simulink model "JointSpaceControl_BestInertia"  (R2013a)
settings: Solver=ode3  StartTime=0.0  StopTime=sim_end  FixedStep=0.004  MaxStep=0.008  RelTol=1e-3
PreLoadFcn:
  | Initialization
InitFcn:
  | Initialization
values from neighbouring files (symbols this model uses):
  a_max = [27 27 27 27 27 27]    [Initialization.m]
  dq_0 = qd_actual.signals.values(1,:)    [Initialization.m]
  K_0 = [K0_11, zeros(3,3); zeros(3,3),omega_P_small^2*eye(3,3)]    [Initialization.m]    (also in Plot_PD_Estimation.m)
  K_1 = [K1_11, zeros(3,3); zeros(3,3),2*omega_D_small*eye(3,3)]    [Initialization.m]    (also in Plot_PD_Estimation.m)
  q_0 = q_actual.signals.values(1,:)    [Initialization.m]
  q_max = 2*pi*ones(1,6)    [Initialization.m]
  q_min = -2*pi*ones(1,6)    [Initialization.m]
  torque_max = [150 150 150 28 28 28]    [Initialization.m]
  v_max = 3.4*ones(1,6)    [Initialization.m]
libraries: dsparch4 x30, simulink x2
(part 1 of 3)
settings Model: Creator=kasiunia  LastModifiedBy=kasiunia

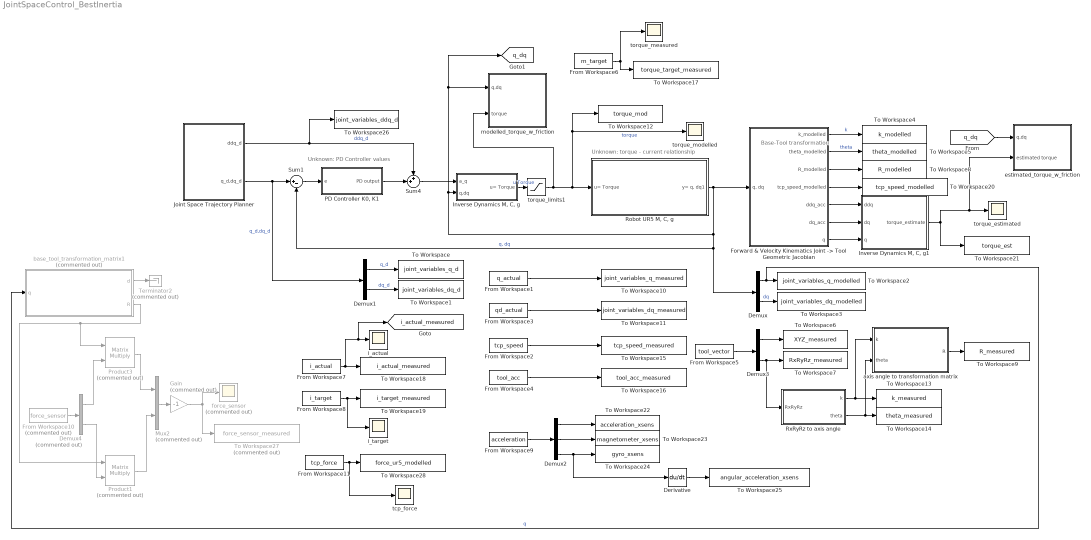
== system JointSpaceControl_BestInertia ==
  note: Base-Tool transformation
  note: Unknown: torque - current relationship
  note: Unknown: PD Controller values
  Demux : Demux  Outputs=[6 6]
  Demux1 : Demux  Outputs=[6 6]
  Demux2 : Demux  Outputs=[3 3 3]
  Demux3 : Demux  Outputs=[3 3]
  Demux4 : Demux  Commented=on  Outputs=[3 3 ]
  Derivative : Derivative
  "Forward & Velocity Kinematics Joint -> Tool Geometric Jacobian" : Subsystem
  From Workspace1 : FromWorkspace  VariableName=q_actual  SampleTime=0  OutputAfterFinalValue=Holding final value
  From Workspace10 : FromWorkspace  Commented=on  VariableName=force_sensor  SampleTime=0  OutputAfterFinalValue=Holding final value
  From Workspace11 : FromWorkspace  VariableName=tcp_force  SampleTime=0  OutputAfterFinalValue=Holding final value
  From Workspace2 : FromWorkspace  VariableName=tcp_speed  SampleTime=0  OutputAfterFinalValue=Setting to zero
  From Workspace3 : FromWorkspace  VariableName=qd_actual  SampleTime=0  OutputAfterFinalValue=Setting to zero
  From Workspace4 : FromWorkspace  VariableName=tool_acc  SampleTime=0  OutputAfterFinalValue=Setting to zero
  From Workspace5 : FromWorkspace  VariableName=tool_vector  SampleTime=0  OutputAfterFinalValue=Holding final value
  From Workspace6 : FromWorkspace  VariableName=m_target  SampleTime=0  OutputAfterFinalValue=Holding final value
  From Workspace7 : FromWorkspace  VariableName=i_actual  SampleTime=0  OutputAfterFinalValue=Holding final value
  From Workspace8 : FromWorkspace  VariableName=i_target  SampleTime=0  OutputAfterFinalValue=Holding final value
  From Workspace9 : FromWorkspace  VariableName=acceleration  SampleTime=0  OutputAfterFinalValue=Setting to zero
  Gain : Gain  Commented=on  Gain=-1
  "Inverse Dynamics M, C, g" : Subsystem
  "Inverse Dynamics M, C, g1" : Subsystem
  Joint Space Trajectory Planner : Subsystem
  Mux2 : Mux  Commented=on  Inputs=[3 3]
  "PD Controller K0, K1" : Subsystem
  Product1 : Product  Commented=on  Multiplication=Matrix(*)
  Product3 : Product  Commented=on  Multiplication=Matrix(*)
  "Robot UR5 M, C, g" : Subsystem
  RxRyRz to axis angle : MATLAB Function  TreatAsAtomicUnit=on
  Sum1 : Sum  Inputs=|+-
  Sum4 : Sum  Inputs=++|
  Terminator2 : Terminator  Commented=on
  To Workspace : ToWorkspace  VariableName=joint_variables_q_d  SampleTime=-1  SaveFormat=Timeseries
  To Workspace1 : ToWorkspace  VariableName=joint_variables_dq_d  SampleTime=-1  SaveFormat=Timeseries
  To Workspace10 : ToWorkspace  VariableName=joint_variables_q_measured  SampleTime=-1  SaveFormat=Timeseries
  To Workspace11 : ToWorkspace  VariableName=joint_variables_dq_measured  SampleTime=-1  SaveFormat=Timeseries
  To Workspace12 : ToWorkspace  VariableName=torque_mod  SampleTime=-1  SaveFormat=Timeseries
  To Workspace13 : ToWorkspace  VariableName=k_measured  SampleTime=-1  SaveFormat=Timeseries
  To Workspace14 : ToWorkspace  VariableName=theta_measured  SampleTime=-1  SaveFormat=Timeseries
  To Workspace15 : ToWorkspace  VariableName=tcp_speed_measured  SampleTime=-1  SaveFormat=Timeseries
  To Workspace16 : ToWorkspace  VariableName=tool_acc_measured  SampleTime=-1  SaveFormat=Timeseries
  To Workspace17 : ToWorkspace  VariableName=torque_target_measured  SampleTime=-1  SaveFormat=Timeseries
  To Workspace18 : ToWorkspace  VariableName=i_actual_measured  SampleTime=-1  SaveFormat=Timeseries
  To Workspace19 : ToWorkspace  VariableName=i_target_measured  SampleTime=-1  SaveFormat=Timeseries
  To Workspace2 : ToWorkspace  VariableName=joint_variables_q_modelled  SampleTime=-1  SaveFormat=Timeseries
  To Workspace20 : ToWorkspace  VariableName=tcp_speed_modelled  SampleTime=-1  SaveFormat=Timeseries
  To Workspace21 : ToWorkspace  VariableName=torque_est  SampleTime=-1  SaveFormat=Timeseries
  To Workspace22 : ToWorkspace  VariableName=acceleration_xsens  SampleTime=-1  SaveFormat=Timeseries
  To Workspace23 : ToWorkspace  VariableName=magnetometer_xsens  SampleTime=-1  SaveFormat=Timeseries
  To Workspace24 : ToWorkspace  VariableName=gyro_xsens  SampleTime=-1  SaveFormat=Timeseries
  To Workspace25 : ToWorkspace  VariableName=angular_acceleration_xsens  SampleTime=-1  SaveFormat=Timeseries
  To Workspace26 : ToWorkspace  VariableName=joint_variables_ddq_d  SampleTime=-1  SaveFormat=Timeseries
  To Workspace27 : ToWorkspace  Commented=on  VariableName=force_sensor_measured  SampleTime=-1  SaveFormat=Timeseries
  To Workspace28 : ToWorkspace  VariableName=force_ur5_modelled  SampleTime=-1  SaveFormat=Timeseries
  To Workspace3 : ToWorkspace  VariableName=joint_variables_dq_modelled  SampleTime=-1  SaveFormat=Timeseries
  To Workspace4 : ToWorkspace  VariableName=k_modelled  SampleTime=-1  SaveFormat=Timeseries
  To Workspace5 : ToWorkspace  VariableName=theta_modelled  SampleTime=-1  SaveFormat=Timeseries
  To Workspace6 : ToWorkspace  VariableName=XYZ_measured  SampleTime=-1  SaveFormat=Timeseries
  To Workspace7 : ToWorkspace  VariableName=RxRyRz_measured  SampleTime=-1  SaveFormat=Timeseries
  To Workspace8 : ToWorkspace  VariableName=R_modelled  SampleTime=-1  SaveFormat=Timeseries
  To Workspace9 : ToWorkspace  VariableName=R_measured  SampleTime=-1  SaveFormat=Timeseries
  axis angle to transformation matrix : MATLAB Function  TreatAsAtomicUnit=on
  base_tool_transformation_matrix1 : MATLAB Function  Commented=on  TreatAsAtomicUnit=on
  estimated_torque_w_friction : Subsystem
  force_sensor : Scope  Commented=on
      settings: ShowLegends=on  SaveName=ScopeData19
  i_actual : Scope
      settings: ShowLegends=on  TimeRange=25  YMin=-10  YMax=15  SaveName=ScopeData12
  i_target : Scope
      settings: SaveName=ScopeData13
  modelled_torque_w_friction : Subsystem
  tcp_force : Scope
      settings: SaveName=ScopeData20
  torque_estimated : Scope
      settings: ShowLegends=on  TimeRange=30  YMin=-2250  YMax=2250  SaveName=ScopeData15
  torque_limits1 : Saturate  UpperLimit=torque_max  LowerLimit=-torque_max
  torque_measured : Scope
      settings: ShowLegends=on  TimeRange=20.1629  YMin=-30  YMax=90  SaveName=ScopeData16
  torque_modelled : Scope
      settings: ShowLegends=on  TimeRange=20.1629  YMin=-2.5  YMax=55  SaveName=ScopeData17
  tag scope: i_actual_measured=global, q_dq=global
  wires:
  Joint Space Trajectory Planner/2(q_d,dq_d) -> Sum1/1, Demux1/1  "q_d,dq_d"
  Sum1/1 -> "PD Controller K0, K1"/1(e)
  "Robot UR5 M, C, g"/1("y= q, dq1") -> Sum1/2, Demux/1, [q_dq], modelled_torque_w_friction/1(q,dq), "Inverse Dynamics M, C, g"/2(q,dq), "Forward & Velocity Kinematics Joint -> Tool Geometric Jacobian"/1("q, dq")  "q, dq"
  Joint Space Trajectory Planner/1(ddq_d) -> Sum4/1, To Workspace26/1  "ddq_d"
  Demux1/1 -> To Workspace/1  "q_d"
  Demux1/2 -> To Workspace1/1  "dq_d"
  Demux/1 -> base_tool_transformation_matrix1/1(q), To Workspace2/1  "q"
  Demux/2 -> To Workspace3/1  "dq"
  From Workspace5/1 -> Demux3/1
  Demux3/1 -> To Workspace6/1
  Demux3/2 -> RxRyRz to axis angle/1(RxRyRz), To Workspace7/1
  "Forward & Velocity Kinematics Joint -> Tool Geometric Jacobian"/1(k_modelled) -> To Workspace4/1  "k"
  "Forward & Velocity Kinematics Joint -> Tool Geometric Jacobian"/2(theta_modelled) -> To Workspace5/1  "theta"
  RxRyRz to axis angle/1(k) -> axis angle to transformation matrix/1(k), To Workspace13/1
  RxRyRz to axis angle/2(theta) -> axis angle to transformation matrix/2(theta), To Workspace14/1
  "Forward & Velocity Kinematics Joint -> Tool Geometric Jacobian"/3(R_modelled) -> To Workspace8/1
  axis angle to transformation matrix/1(R) -> To Workspace9/1
  From Workspace2/1 -> To Workspace15/1
  From Workspace4/1 -> To Workspace16/1
  From Workspace6/1 -> torque_measured/1, To Workspace17/1
  From Workspace7/1 -> [i_actual_measured], i_actual/1, To Workspace18/1
  From Workspace8/1 -> i_target/1, To Workspace19/1
  "Forward & Velocity Kinematics Joint -> Tool Geometric Jacobian"/4(tcp_speed_modelled) -> To Workspace20/1
  "Forward & Velocity Kinematics Joint -> Tool Geometric Jacobian"/5(ddq_acc) -> "Inverse Dynamics M, C, g1"/1(ddq)
  "Forward & Velocity Kinematics Joint -> Tool Geometric Jacobian"/6(dq_acc) -> "Inverse Dynamics M, C, g1"/2(dq)
  "Inverse Dynamics M, C, g1"/1(torque_estimate) -> To Workspace21/1, estimated_torque_w_friction/2(estimated torque), torque_estimated/1
  "Forward & Velocity Kinematics Joint -> Tool Geometric Jacobian"/7(q) -> "Inverse Dynamics M, C, g1"/3(q)
  From Workspace9/1 -> Demux2/1
  Demux2/1 -> To Workspace22/1
  Demux2/2 -> To Workspace23/1
  Demux2/3 -> To Workspace24/1, Derivative/1
  Derivative/1 -> To Workspace25/1
  "Inverse Dynamics M, C, g"/1(u= Torque) -> torque_limits1/1  "u Torque"
  torque_limits1/1 -> modelled_torque_w_friction/2(torque), torque_modelled/1, To Workspace12/1, "Robot UR5 M, C, g"/1(u= Torque)  "torque"
  From Workspace1/1 -> To Workspace10/1
  From Workspace3/1 -> To Workspace11/1
  From Workspace11/1 -> tcp_force/1, To Workspace28/1
  [q_dq] -> estimated_torque_w_friction/1(q,dq)
  "PD Controller K0, K1"/1(PD output) -> Sum4/2
  Sum4/1 -> "Inverse Dynamics M, C, g"/1(a_q)
  base_tool_transformation_matrix1/1(d) -> Terminator2/1
  base_tool_transformation_matrix1/2(R) -> Product1/1, Product3/1
  From Workspace10/1 -> Demux4/1
  Mux2/1 -> Gain/1
  Product3/1 -> Mux2/1
  Demux4/2 -> Product1/2
  Demux4/1 -> Product3/2
  Product1/1 -> Mux2/2
  Gain/1 -> force_sensor/1, To Workspace27/1

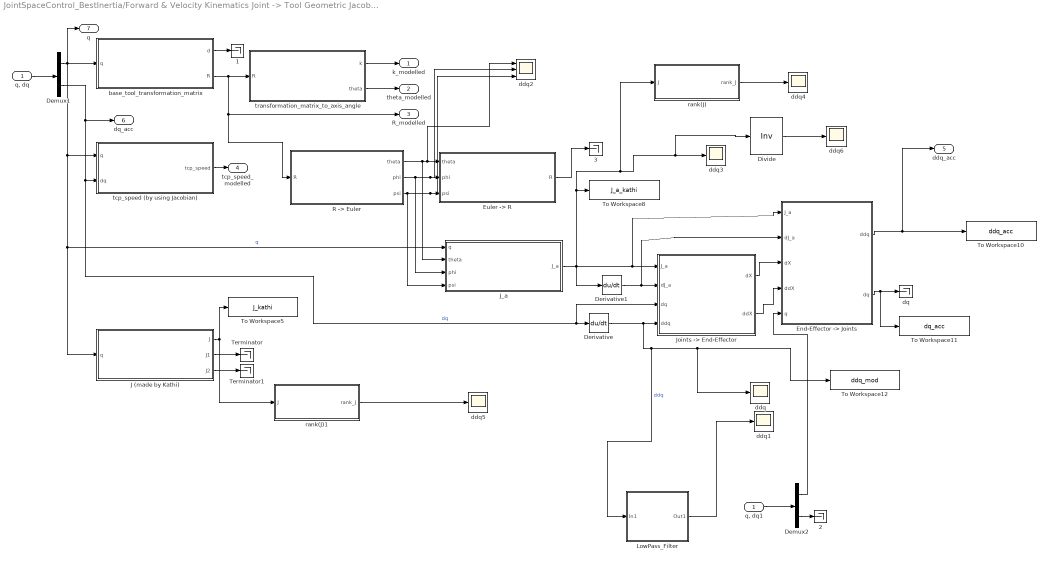
== system JointSpaceControl_BestInertia/Forward & Velocity Kinematics Joint -> Tool Geometric Jacobian ==
  "q, dq" : Inport
  1 : Terminator
  2 : Terminator
  3 : Terminator
  Demux1 : Demux  Outputs=[6 6]
  Demux2 : Demux  Outputs=[6 6]
  Derivative : Derivative
  Derivative1 : Derivative
  Divide : Product  Inputs=/  Multiplication=Matrix(*)
  "End-Effector -> Joints" : Subsystem
  "Euler -> R" : MATLAB Function  TreatAsAtomicUnit=on
  J (made by Kathi) : MATLAB Function  TreatAsAtomicUnit=on
  J_a : MATLAB Function  TreatAsAtomicUnit=on
  "Joints -> End-Effector" : Subsystem
  LowPass_Filter : Subsystem
  "R -> Euler" : MATLAB Function  TreatAsAtomicUnit=on
  Terminator : Terminator
  Terminator1 : Terminator
  To Workspace10 : ToWorkspace  VariableName=ddq_acc  SampleTime=-1  SaveFormat=Timeseries
  To Workspace11 : ToWorkspace  VariableName=dq_acc  SampleTime=-1  SaveFormat=Timeseries
  To Workspace12 : ToWorkspace  VariableName=ddq_mod  SampleTime=-1  SaveFormat=Timeseries
  To Workspace5 : ToWorkspace  VariableName=J_kathi  SampleTime=-1  SaveFormat=Timeseries
  To Workspace8 : ToWorkspace  VariableName=J_a_kathi  SampleTime=-1  SaveFormat=Timeseries
  base_tool_transformation_matrix : MATLAB Function  TreatAsAtomicUnit=on
  ddq{,1,3..6} (6 alike) : Scope
      ddq settings: ShowLegends=on  SaveName=ScopeData7
      ddq1 settings: ShowLegends=on  SaveName=ScopeData35
      ddq3 settings: ShowLegends=on  SaveName=ScopeData5
      ddq4 settings: ShowLegends=on  SaveName=ScopeData9
      ddq5 settings: ShowLegends=on  SaveName=ScopeData10
      ddq6 settings: ShowLegends=on  SaveName=ScopeData11
  ddq2 : Scope  NumInputPorts=3
      settings: ShowLegends=on  YMin=-5~-5~-5  YMax=5~5~5
  dq : Terminator
  "q, dq1" : InportShadow
  rank(J) : MATLAB Function  TreatAsAtomicUnit=on
  rank(J)1 : MATLAB Function  TreatAsAtomicUnit=on
  tcp_speed (by using Jacobian) : MATLAB Function  TreatAsAtomicUnit=on
  transformation_matrix_to_axis_angle : MATLAB Function  TreatAsAtomicUnit=on
  k_modelled : Outport
  theta_modelled : Outport  Port=2
  R_modelled : Outport  Port=3
  tcp_speed_modelled : Outport  Port=4
  ddq_acc : Outport  Port=5
  dq_acc : Outport  Port=6
  q : Outport  Port=7
  wires:
  "q, dq"/1 -> Demux1/1
  Demux1/1 -> q/1, J (made by Kathi)/1(q), J_a/1(q), tcp_speed (by using Jacobian)/1(q), base_tool_transformation_matrix/1(q)  "q"
  Demux1/2 -> dq_acc/1, "Joints -> End-Effector"/3(dq), Derivative/1, tcp_speed (by using Jacobian)/2(dq)  "dq"
  base_tool_transformation_matrix/2(R) -> transformation_matrix_to_axis_angle/1(R), "R -> Euler"/1(R), R_modelled/1
  transformation_matrix_to_axis_angle/1(k) -> k_modelled/1
  transformation_matrix_to_axis_angle/2(theta) -> theta_modelled/1
  J (made by Kathi)/1(J) -> To Workspace5/1, rank(J)1/1(J)
  tcp_speed (by using Jacobian)/1(tcp_speed) -> tcp_speed_modelled/1
  "R -> Euler"/3(psi) -> J_a/4(psi), ddq2/3, "Euler -> R"/3(psi)
  "R -> Euler"/2(phi) -> J_a/3(phi), ddq2/2, "Euler -> R"/2(phi)
  "R -> Euler"/1(theta) -> J_a/2(theta), ddq2/1, "Euler -> R"/1(theta)
  base_tool_transformation_matrix/1(d) -> 1/1
  J_a/1(J_a) -> "Joints -> End-Effector"/1(J_a), "End-Effector -> Joints"/1(J_a), rank(J)/1(J), Divide/1, ddq3/1, To Workspace8/1, Derivative1/1
  Derivative/1 -> "Joints -> End-Effector"/4(ddq), LowPass_Filter/1(In1), ddq/1, To Workspace12/1  "ddq"
  "Joints -> End-Effector"/2(ddX) -> "End-Effector -> Joints"/4(ddX)
  "Joints -> End-Effector"/1(dX) -> "End-Effector -> Joints"/3(dX)
  Derivative1/1 -> "Joints -> End-Effector"/2(dJ_a), "End-Effector -> Joints"/2(dJ_a)
  "End-Effector -> Joints"/2(dq) -> To Workspace11/1, dq/1
  J (made by Kathi)/2(J1) -> Terminator/1
  J (made by Kathi)/3(J2) -> Terminator1/1
  "End-Effector -> Joints"/1(ddq) -> ddq_acc/1, To Workspace10/1
  "q, dq1"/1 -> Demux2/1
  Demux2/2 -> 2/1
  Demux2/1 -> "End-Effector -> Joints"/5(q)
  "Euler -> R"/1(R) -> 3/1
  LowPass_Filter/1(Out1) -> ddq1/1
  rank(J)/1(rank_J) -> ddq4/1
  rank(J)1/1(rank_J) -> ddq5/1
  Divide/1 -> ddq6/1

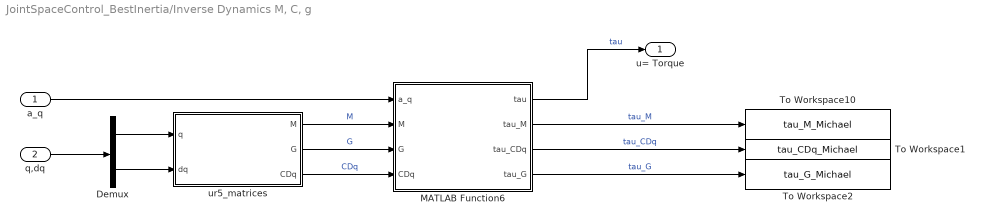
== system JointSpaceControl_BestInertia/Inverse Dynamics M, C, g ==
  a_q : Inport
  q,dq : Inport  Port=2
  Demux : Demux  Outputs=[6 6]
  MATLAB Function6 : MATLAB Function  TreatAsAtomicUnit=on
  To Workspace1 : ToWorkspace  VariableName=tau_CDq_Michael  SampleTime=-1  SaveFormat=Timeseries
  To Workspace10 : ToWorkspace  VariableName=tau_M_Michael  SampleTime=-1  SaveFormat=Timeseries
  To Workspace2 : ToWorkspace  VariableName=tau_G_Michael  SampleTime=-1  SaveFormat=Timeseries
  ur5_matrices : MATLAB Function  TreatAsAtomicUnit=on
  u= Torque : Outport
  wires:
  ur5_matrices/1(M) -> MATLAB Function6/2(M)  "M"
  ur5_matrices/3(CDq) -> MATLAB Function6/4(CDq)  "CDq"
  a_q/1 -> MATLAB Function6/1(a_q)
  Demux/1 -> ur5_matrices/1(q)
  Demux/2 -> ur5_matrices/2(dq)
  q,dq/1 -> Demux/1
  MATLAB Function6/1(tau) -> u= Torque/1  "tau"
  MATLAB Function6/2(tau_M) -> To Workspace10/1  "tau_M"
  MATLAB Function6/3(tau_CDq) -> To Workspace1/1  "tau_CDq"
  MATLAB Function6/4(tau_G) -> To Workspace2/1  "tau_G"
  ur5_matrices/2(G) -> MATLAB Function6/3(G)  "G"

== system JointSpaceControl_BestInertia/Inverse Dynamics M, C, g1 ==
  ddq : Inport
  dq : Inport  Port=2
  q : Inport  Port=3
  ur5_invDynamics : MATLAB Function  TreatAsAtomicUnit=on
  ur5_matrices : MATLAB Function  TreatAsAtomicUnit=on
  torque_estimate : Outport
  wires:
  ur5_invDynamics/1(tau) -> torque_estimate/1  "tau"
  ddq/1 -> ur5_invDynamics/1(a_q)
  ur5_matrices/3(CDq) -> ur5_invDynamics/4(CDq)
  ur5_matrices/2(G) -> ur5_invDynamics/3(G)
  ur5_matrices/1(M) -> ur5_invDynamics/2(M)
  q/1 -> ur5_matrices/1(q)
  dq/1 -> ur5_matrices/2(dq)

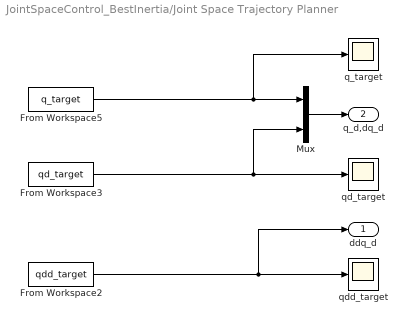
== system JointSpaceControl_BestInertia/Joint Space Trajectory Planner ==
  From Workspace2 : FromWorkspace  VariableName=qdd_target  SampleTime=0  OutputAfterFinalValue=Setting to zero
  From Workspace3 : FromWorkspace  VariableName=qd_target  SampleTime=0  OutputAfterFinalValue=Setting to zero
  From Workspace5 : FromWorkspace  VariableName=q_target  SampleTime=0  OutputAfterFinalValue=Holding final value
  Mux : Mux  Inputs=[6 6]
  q_target : Scope
      settings: ShowLegends=on
  qd_target : Scope
      settings: ShowLegends=on  SaveName=ScopeData2
  qdd_target : Scope
      settings: ShowLegends=on  SaveName=ScopeData3
  ddq_d : Outport
  q_d,dq_d : Outport  Port=2
  wires:
  Mux/1 -> q_d,dq_d/1
  From Workspace5/1 -> Mux/1, q_target/1
  From Workspace3/1 -> Mux/2, qd_target/1
  From Workspace2/1 -> ddq_d/1, qdd_target/1

== system JointSpaceControl_BestInertia/PD Controller K0, K1 ==
  e : Inport
  Demux : Demux  Outputs=[6 6]
  Gain : Gain  Gain=K_0  Multiplication=Matrix(K*u) (u vector)
  Gain1 : Gain  Gain=K_1  Multiplication=Matrix(K*u) (u vector)
  Sum : Sum  Inputs=|++
  PD output : Outport
  wires:
  e/1 -> Demux/1
  Sum/1 -> PD output/1
  Demux/1 -> Gain/1  "e_q = q_d - q"
  Demux/2 -> Gain1/1  "e_dq = dq_d - dq"
  Gain1/1 -> Sum/2
  Gain/1 -> Sum/1

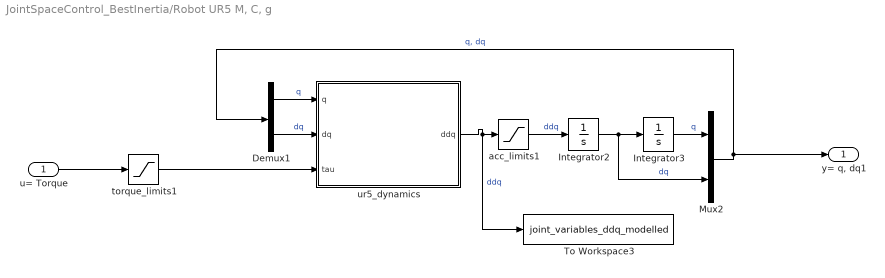
== system JointSpaceControl_BestInertia/Robot UR5 M, C, g ==
  u= Torque : Inport
  Demux1 : Demux  Outputs=[6 6]
  Integrator2 : Integrator  InitialCondition=[dq_0]  LimitOutput=on  UpperSaturationLimit=v_max  LowerSaturationLimit=-v_max  ContinuousStateAttributes='velocity'
  Integrator3 : Integrator  InitialCondition=[q_0]  LimitOutput=on  UpperSaturationLimit=q_max  LowerSaturationLimit=q_min  ContinuousStateAttributes='position'
  Mux2 : Mux  Inputs=[6 6]
  To Workspace3 : ToWorkspace  VariableName=joint_variables_ddq_modelled  SampleTime=-1  SaveFormat=Timeseries
  acc_limits1 : Saturate  UpperLimit=a_max  LowerLimit=-a_max
  torque_limits1 : Saturate  UpperLimit=torque_max  LowerLimit=-torque_max
  ur5_dynamics : MATLAB Function  TreatAsAtomicUnit=on
  "y= q, dq1" : Outport
  wires:
  ur5_dynamics/1(ddq) -> To Workspace3/1, acc_limits1/1  "ddq"
  Integrator2/1 -> Integrator3/1, Mux2/2  "dq"
  Integrator3/1 -> Mux2/1  "q"
  Mux2/1 -> "y= q, dq1"/1, Demux1/1  "q, dq"
  Demux1/1 -> ur5_dynamics/1(q)  "q"
  Demux1/2 -> ur5_dynamics/2(dq)  "dq"
  acc_limits1/1 -> Integrator2/1  "ddq"
  torque_limits1/1 -> ur5_dynamics/3(tau)
  u= Torque/1 -> torque_limits1/1

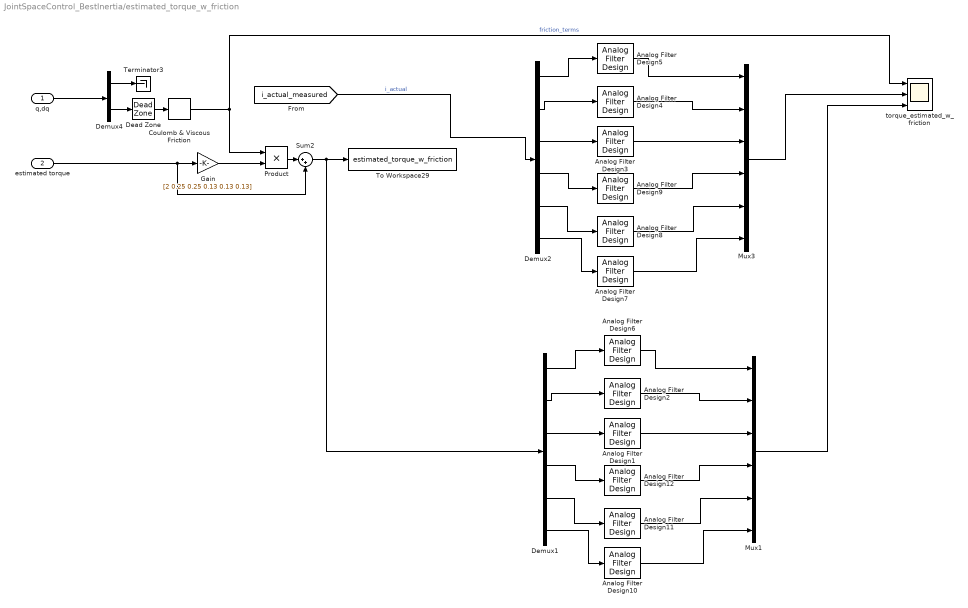
== system JointSpaceControl_BestInertia/estimated_torque_w_friction ==
  q,dq : Inport
  estimated torque : Inport  Port=2
  Analog Filter Design{1..12} (12 alike) : dsparch4/Analog Filter Design  method=Butterworth  filttype=Lowpass  N=10  Wlo=30  Whi=80  Rp=2  Rs=40
  Coulomb & Viscous Friction : simulink/Discontinuities/Coulomb & Viscous Friction  offset=1  gain=1
  Dead Zone : DeadZone  LowerValue=-0.02  UpperValue=0.02  SaturateOnIntegerOverflow=on
  Demux1 : Demux  Outputs=[1 1 1 1 1 1]
  Demux2 : Demux  Outputs=[1 1 1 1 1 1]
  Demux4 : Demux  Outputs=[6 6]
  Gain : Gain  Gain=[2 0.25 0.25 0.13 0.13 0.13]
  Mux1 : Mux  Inputs=[1 1 1 1 1 1]
  Mux3 : Mux  Inputs=[1 1 1 1 1 1]
  Product : Product
  Sum2 : Sum  Inputs=|++
  Terminator3 : Terminator
  To Workspace29 : ToWorkspace  VariableName=estimated_torque_w_friction  SampleTime=-1  SaveFormat=Timeseries
  torque_estimated_w_friction : Scope  NumInputPorts=3
      settings: ShowLegends=on  TimeRange=25  YMin=-2.25~-2~-40  YMax=2.25~6.5~80  SaveName=ScopeData18
  wires:
  estimated torque/1 -> Gain/1, Sum2/2
  q,dq/1 -> Demux4/1
  Demux4/2 -> Dead Zone/1
  Product/1 -> Sum2/1
  Dead Zone/1 -> Coulomb & Viscous Friction/1
  Sum2/1 -> Demux1/1, To Workspace29/1
  Gain/1 -> Product/2
  Coulomb & Viscous Friction/1 -> torque_estimated_w_friction/1, Product/1  "friction_terms"
  Demux4/1 -> Terminator3/1
  Demux2/1 -> Analog Filter Design5/1
  Demux2/2 -> Analog Filter Design4/1
  Demux2/3 -> Analog Filter Design3/1
  Analog Filter Design5/1 -> Mux3/1
  Analog Filter Design4/1 -> Mux3/2
  Analog Filter Design3/1 -> Mux3/3
  [i_actual_measured] -> Demux2/1  "i_actual"
  Mux3/1 -> torque_estimated_w_friction/2
  Demux2/4 -> Analog Filter Design9/1
  Demux2/5 -> Analog Filter Design8/1
  Demux2/6 -> Analog Filter Design7/1
  Analog Filter Design9/1 -> Mux3/4
  Analog Filter Design8/1 -> Mux3/5
  Analog Filter Design7/1 -> Mux3/6
  Demux1/1 -> Analog Filter Design6/1
  Demux1/2 -> Analog Filter Design2/1
  Demux1/3 -> Analog Filter Design1/1
  Analog Filter Design6/1 -> Mux1/1
  Analog Filter Design2/1 -> Mux1/2
  Analog Filter Design1/1 -> Mux1/3
  Demux1/4 -> Analog Filter Design12/1
  Demux1/5 -> Analog Filter Design11/1
  Demux1/6 -> Analog Filter Design10/1
  Analog Filter Design12/1 -> Mux1/4
  Analog Filter Design11/1 -> Mux1/5
  Analog Filter Design10/1 -> Mux1/6
  Mux1/1 -> torque_estimated_w_friction/3

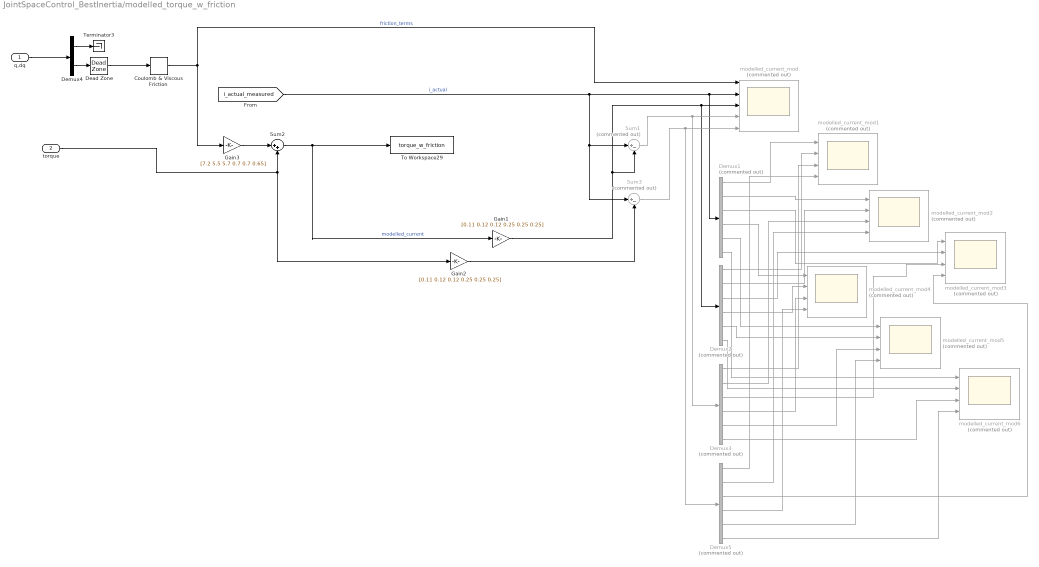
== system JointSpaceControl_BestInertia/modelled_torque_w_friction ==
  q,dq : Inport
  torque : Inport  Port=2
  Coulomb & Viscous Friction : simulink/Discontinuities/Coulomb & Viscous Friction  offset=1  gain=1
  Dead Zone : DeadZone  LowerValue=-0.02  UpperValue=0.02  SaturateOnIntegerOverflow=on
  Demux{1..3,5} (4 alike) : Demux  Commented=on  Outputs=[1 1 1 1 1 1]
  Demux4 : Demux  Outputs=[6 6]
  Gain1 : Gain  Gain=[0.11 0.12 0.12 0.25 0.25 0.25]
  Gain2 : Gain  Gain=[0.11 0.12 0.12 0.25 0.25 0.25]
  Gain3 : Gain  Gain=[7.2 5.5 5.7 0.7 0.7 0.65]
  Sum1 : Sum  Commented=on  Inputs=|+-
  Sum2 : Sum  Inputs=|++
  Sum3 : Sum  Commented=on  Inputs=|+-
  Terminator3 : Terminator
  To Workspace29 : ToWorkspace  VariableName=torque_w_friction  SampleTime=-1  SaveFormat=Timeseries
  modelled_current_mod : Scope  Commented=on  NumInputPorts=5
      settings: ShowLegends=on  TimeRange=15.704  YMin=-2.5~-2.5~-5~-5~-5  YMax=2.25~7.5~60~5~5  SaveName=ScopeData18
  modelled_current_mod{1..6} (6 alike) : Scope  Commented=on  NumInputPorts=4
      modelled_current_mod1 settings: ShowLegends=on  TimeRange=15.704  YMin=-2.5~-2.5~-5~-5  YMax=2.25~7.5~60~5  SaveName=ScopeData27
      modelled_current_mod2 settings: ShowLegends=on  TimeRange=15.704  YMin=-2.5~-2.5~-5~-5  YMax=2.25~7.5~60~5  SaveName=ScopeData28
      modelled_current_mod3 settings: ShowLegends=on  TimeRange=15.704  YMin=-2.5~-2.5~-5~-5  YMax=2.25~7.5~60~5  SaveName=ScopeData30
      modelled_current_mod4 settings: ShowLegends=on  TimeRange=15.704  YMin=-2.5~-2.5~-5~-5  YMax=2.25~7.5~60~5  SaveName=ScopeData31
      modelled_current_mod5 settings: ShowLegends=on  TimeRange=15.704  YMin=-2.5~-2.5~-5~-5  YMax=2.25~7.5~60~5  SaveName=ScopeData32
      modelled_current_mod6 settings: ShowLegends=on  TimeRange=15.704  YMin=-2.5~-2.5~-5~-5  YMax=2.25~7.5~60~5  SaveName=ScopeData33
  wires:
  [i_actual_measured] -> Sum3/1, Sum1/1, Demux1/1, modelled_current_mod/2  "i_actual"
  Demux4/1 -> Terminator3/1
  Coulomb & Viscous Friction/1 -> Gain3/1, modelled_current_mod/1  "friction_terms"
  Sum2/1 -> Gain1/1, To Workspace29/1  "modelled_current"
  Dead Zone/1 -> Coulomb & Viscous Friction/1
  Demux4/2 -> Dead Zone/1
  q,dq/1 -> Demux4/1
  Gain1/1 -> Sum1/2, Demux2/1, modelled_current_mod/3
  Sum1/1 -> Demux3/1, modelled_current_mod/4
  Sum3/1 -> Demux5/1, modelled_current_mod/5
  torque/1 -> Gain2/1, Sum2/2
  Gain2/1 -> Sum3/2
  Demux1/1 -> modelled_current_mod1/1
  Demux1/2 -> modelled_current_mod2/1
  Demux1/3 -> modelled_current_mod3/1
  Demux1/4 -> modelled_current_mod4/1
  Demux1/5 -> modelled_current_mod5/1
  Demux1/6 -> modelled_current_mod6/1
  Demux2/1 -> modelled_current_mod1/2
  Demux2/2 -> modelled_current_mod2/2
  Demux2/3 -> modelled_current_mod3/2
  Demux2/4 -> modelled_current_mod4/2
  Demux2/5 -> modelled_current_mod5/2
  Demux2/6 -> modelled_current_mod6/2
  Demux3/1 -> modelled_current_mod1/3
  Demux3/2 -> modelled_current_mod2/3
  Demux3/3 -> modelled_current_mod3/3
  Demux3/4 -> modelled_current_mod4/3
  Demux3/5 -> modelled_current_mod5/3
  Demux3/6 -> modelled_current_mod6/3
  Demux5/1 -> modelled_current_mod1/4
  Demux5/2 -> modelled_current_mod2/4
  Demux5/3 -> modelled_current_mod3/4
  Demux5/4 -> modelled_current_mod4/4
  Demux5/5 -> modelled_current_mod5/4
  Demux5/6 -> modelled_current_mod6/4
  Gain3/1 -> Sum2/1

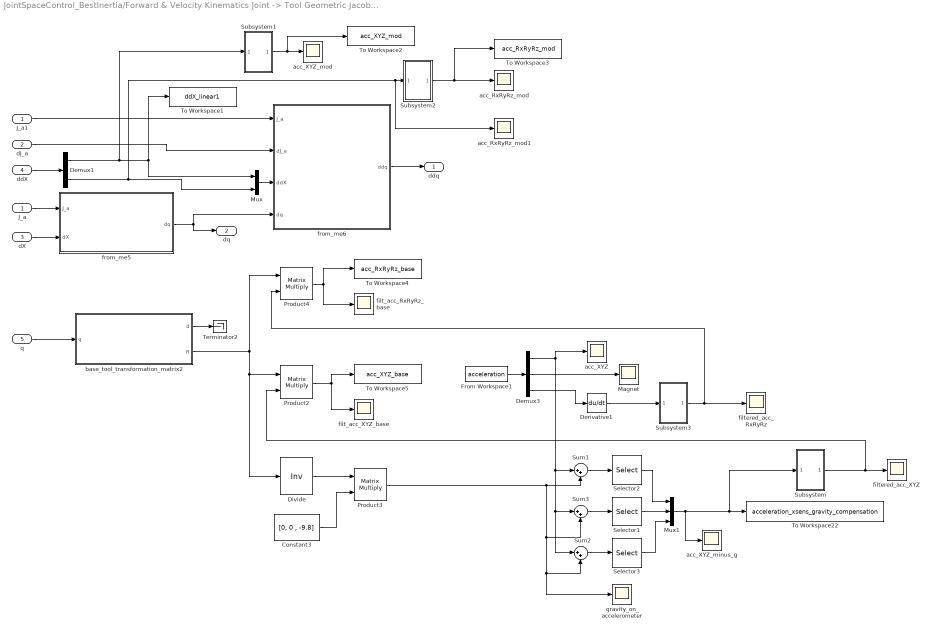
== system JointSpaceControl_BestInertia/Forward & Velocity Kinematics Joint -> Tool Geometric Jacobian/End-Effector -> Joints ==
  J_a : Inport
  dJ_a : Inport  Port=2
  dX : Inport  Port=3
  ddX : Inport  Port=4
  q : Inport  Port=5
  Constant3 : Constant  Value=[0, 0 , -9.8]
  Demux1 : Demux  Outputs=[3 3]
  Demux3 : Demux  Outputs=[3 3 3]
  Derivative1 : Derivative
  Divide : Product  Inputs=/  Multiplication=Matrix(*)
  From Workspace1 : FromWorkspace  VariableName=acceleration  SampleTime=0  OutputAfterFinalValue=Setting to zero
  J_a1 : InportShadow
  Magnet : Scope
      settings: ShowLegends=on  SaveName=ScopeData22
  Mux : Mux  Inputs=[3 3]
  Mux1 : Mux  Inputs=[1 1 1]
  Product2 : Product  Multiplication=Matrix(*)
  Product3 : Product  Multiplication=Matrix(*)
  Product4 : Product  Multiplication=Matrix(*)
  Selector1 : Selector  InputPortWidth=3  IndexOptions=Index vector (dialog)  Indices=[2]  OutputSizes=1
  Selector2 : Selector  InputPortWidth=3  IndexOptions=Index vector (dialog)  Indices=[1]  OutputSizes=1
  Selector3 : Selector  InputPortWidth=3  IndexOptions=Index vector (dialog)  Indices=[3]  OutputSizes=1
  Subsystem : Subsystem
  Subsystem1 : Subsystem
  Subsystem2 : Subsystem
  Subsystem3 : Subsystem
  Sum1 : Sum  Inputs=|++
  Sum2 : Sum  Inputs=|++
  Sum3 : Sum  Inputs=|++
  Terminator2 : Terminator
  To Workspace1 : ToWorkspace  VariableName=ddX_linear1  SampleTime=-1  SaveFormat=Timeseries
  To Workspace2 : ToWorkspace  VariableName=acc_XYZ_mod  SampleTime=-1  SaveFormat=Timeseries
  To Workspace22 : ToWorkspace  VariableName=acceleration_xsens_gravity_compensation  SampleTime=-1  SaveFormat=Timeseries
  To Workspace3 : ToWorkspace  VariableName=acc_RxRyRz_mod  SampleTime=-1  SaveFormat=Timeseries
  To Workspace4 : ToWorkspace  VariableName=acc_RxRyRz_base  SampleTime=-1  SaveFormat=Timeseries
  To Workspace5 : ToWorkspace  VariableName=acc_XYZ_base  SampleTime=-1  SaveFormat=Timeseries
  acc_RxRyRz_mod : Scope
      settings: ShowLegends=on  YMin=-3  YMax=3.5  SaveName=ScopeData34
  acc_RxRyRz_mod1 : Scope
      settings: ShowLegends=on  YMin=-3  YMax=3.5  SaveName=ScopeData6
  acc_XYZ : Scope
      settings: ShowLegends=on  YMin=-10  YMax=17.5  SaveName=ScopeData23
  acc_XYZ_minus_g : Scope
      settings: ShowLegends=on  YMin=-2.25  YMax=3  SaveName=ScopeData24
  acc_XYZ_mod : Scope
      settings: ShowLegends=on  YMin=-3  YMax=3.5  SaveName=ScopeData4
  base_tool_transformation_matrix2 : MATLAB Function  TreatAsAtomicUnit=on
  filt_acc_RxRyRz_base : Scope
      settings: ShowLegends=on  YMin=-3  YMax=3.5  SaveName=ScopeData21
  filt_acc_XYZ_base : Scope
      settings: ShowLegends=on  YMin=-3  YMax=3.5  SaveName=ScopeData8
  filtered_acc_RxRyRz : Scope
      settings: ShowLegends=on  SaveName=ScopeData29
  filtered_acc_XYZ : Scope
      settings: ShowLegends=on  YMin=-3  YMax=3.5  SaveName=ScopeData25
  from_me5 : MATLAB Function  TreatAsAtomicUnit=on
  from_me6 : MATLAB Function  TreatAsAtomicUnit=on
  gravity_on_accelerometer : Scope
      settings: ShowLegends=on  YMin=-6  YMax=9  SaveName=ScopeData14
  ddq : Outport
  dq : Outport  Port=2
  wires:
  from_me6/1(ddq) -> ddq/1
  J_a/1 -> from_me5/1(J_a)
  J_a1/1 -> from_me6/1(J_a)
  dJ_a/1 -> from_me6/2(dJ_a)
  dX/1 -> from_me5/2(dX)
  from_me5/1(dq) -> dq/1, from_me6/4(dq)
  Mux/1 -> from_me6/3(ddX)
  ddX/1 -> Demux1/1
  From Workspace1/1 -> Demux3/1
  Demux3/2 -> Magnet/1
  Demux3/3 -> Derivative1/1
  Demux3/1 -> Sum3/1, Sum2/1, Sum1/1, acc_XYZ/1
  Mux1/1 -> Subsystem/1(In1), To Workspace22/1, acc_XYZ_minus_g/1
  Sum1/1 -> Selector2/1
  Selector2/1 -> Mux1/1
  Sum2/1 -> Selector3/1
  Sum3/1 -> Selector1/1
  Divide/1 -> Product3/1
  Constant3/1 -> Product3/2
  base_tool_transformation_matrix2/2(R) -> Product4/1, Divide/1, Product2/1
  Product3/1 -> gravity_on_accelerometer/1, Sum2/2, Sum3/2, Sum1/2
  q/1 -> base_tool_transformation_matrix2/1(q)
  Selector1/1 -> Mux1/2
  Selector3/1 -> Mux1/3
  Demux1/1 -> Subsystem1/1(In1), To Workspace1/1, Mux/1
  Demux1/2 -> acc_RxRyRz_mod1/1, Subsystem2/1(In1), Mux/2
  base_tool_transformation_matrix2/1(d) -> Terminator2/1
  Subsystem/1(Out1) -> Product2/2, filtered_acc_XYZ/1
  Subsystem1/1(Out1) -> To Workspace2/1, acc_XYZ_mod/1
  Subsystem2/1(Out1) -> To Workspace3/1, acc_RxRyRz_mod/1
  Product4/1 -> To Workspace4/1, filt_acc_RxRyRz_base/1
  Product2/1 -> To Workspace5/1, filt_acc_XYZ_base/1
  Subsystem3/1(Out1) -> Product4/2, filtered_acc_RxRyRz/1
  Derivative1/1 -> Subsystem3/1(In1)

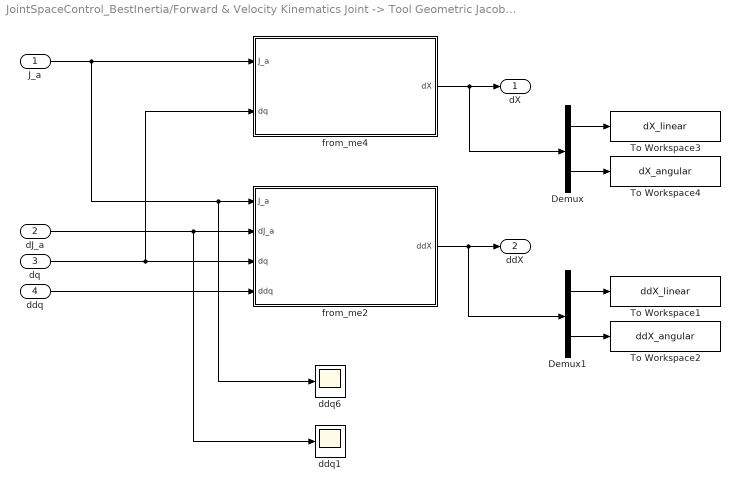
== system JointSpaceControl_BestInertia/Forward & Velocity Kinematics Joint -> Tool Geometric Jacobian/Joints -> End-Effector ==
  J_a : Inport
  dJ_a : Inport  Port=2
  dq : Inport  Port=3
  ddq : Inport  Port=4
  Demux : Demux  Outputs=[3 3]
  Demux1 : Demux  Outputs=[3 3]
  To Workspace1 : ToWorkspace  VariableName=ddX_linear  SampleTime=-1  SaveFormat=Timeseries
  To Workspace2 : ToWorkspace  VariableName=ddX_angular  SampleTime=-1  SaveFormat=Timeseries
  To Workspace3 : ToWorkspace  VariableName=dX_linear  SampleTime=-1  SaveFormat=Timeseries
  To Workspace4 : ToWorkspace  VariableName=dX_angular  SampleTime=-1  SaveFormat=Timeseries
  ddq1 : Scope
      settings: ShowLegends=on  SaveName=ScopeData36
  ddq6 : Scope
      settings: ShowLegends=on  SaveName=ScopeData26
  from_me2 : MATLAB Function  TreatAsAtomicUnit=on
  from_me4 : MATLAB Function  TreatAsAtomicUnit=on
  dX : Outport
  ddX : Outport  Port=2
  wires:
  from_me4/1(dX) -> Demux/1, dX/1
  from_me2/1(ddX) -> Demux1/1, ddX/1
  J_a/1 -> ddq6/1, from_me2/1(J_a), from_me4/1(J_a)
  dJ_a/1 -> ddq1/1, from_me2/2(dJ_a)
  dq/1 -> from_me4/2(dq), from_me2/3(dq)
  ddq/1 -> from_me2/4(ddq)
  Demux/1 -> To Workspace3/1
  Demux/2 -> To Workspace4/1
  Demux1/1 -> To Workspace1/1
  Demux1/2 -> To Workspace2/1

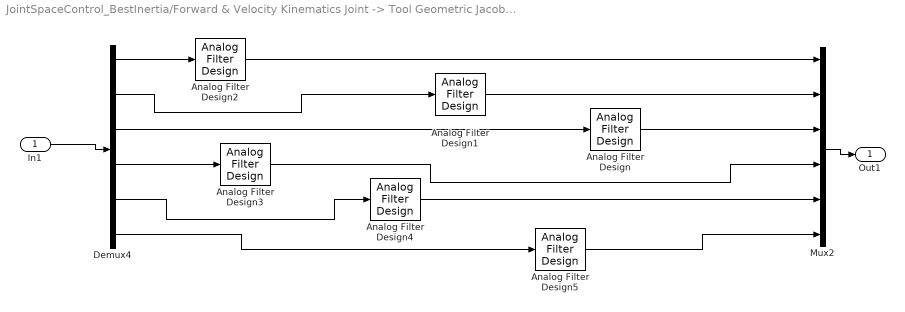
== system JointSpaceControl_BestInertia/Forward & Velocity Kinematics Joint -> Tool Geometric Jacobian/LowPass_Filter ==
  In1 : Inport
  Analog Filter Design{,1..5} (6 alike) : dsparch4/Analog Filter Design  method=Butterworth  filttype=Lowpass  N=3  Wlo=30  Whi=80  Rp=2  Rs=40
  Demux4 : Demux  Outputs=[1 1 1 1 1 1]
  Mux2 : Mux  Inputs=[1 1 1 1 1 1]
  Out1 : Outport
  wires:
  Mux2/1 -> Out1/1
  Analog Filter Design/1 -> Mux2/3
  Analog Filter Design1/1 -> Mux2/2
  Analog Filter Design2/1 -> Mux2/1
  Demux4/3 -> Analog Filter Design/1
  Demux4/2 -> Analog Filter Design1/1
  Demux4/1 -> Analog Filter Design2/1
  In1/1 -> Demux4/1
  Demux4/4 -> Analog Filter Design3/1
  Analog Filter Design3/1 -> Mux2/4
  Demux4/5 -> Analog Filter Design4/1
  Analog Filter Design4/1 -> Mux2/5
  Demux4/6 -> Analog Filter Design5/1
  Analog Filter Design5/1 -> Mux2/6

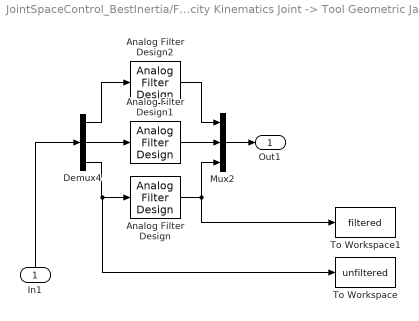
== system JointSpaceControl_BestInertia/Forward & Velocity Kinematics Joint -> Tool Geometric Jacobian/End-Effector -> Joints/Subsystem ==
  In1 : Inport
  Analog Filter Design : dsparch4/Analog Filter Design  method=Butterworth  filttype=Lowpass  N=8  Wlo=30  Whi=80  Rp=2  Rs=40
  Analog Filter Design1 : dsparch4/Analog Filter Design  method=Butterworth  filttype=Lowpass  N=8  Wlo=30  Whi=80  Rp=2  Rs=40
  Analog Filter Design2 : dsparch4/Analog Filter Design  method=Butterworth  filttype=Lowpass  N=8  Wlo=30  Whi=80  Rp=2  Rs=40
  Demux4 : Demux  Outputs=[1 1 1]
  Mux2 : Mux  Inputs=[1 1 1]
  To Workspace : ToWorkspace  VariableName=unfiltered  SampleTime=-1  SaveFormat=Timeseries
  To Workspace1 : ToWorkspace  VariableName=filtered  SampleTime=-1  SaveFormat=Timeseries
  Out1 : Outport
  wires:
  In1/1 -> Demux4/1
  Demux4/1 -> Analog Filter Design2/1
  Demux4/2 -> Analog Filter Design1/1
  Demux4/3 -> To Workspace/1, Analog Filter Design/1
  Analog Filter Design2/1 -> Mux2/1
  Analog Filter Design1/1 -> Mux2/2
  Analog Filter Design/1 -> To Workspace1/1, Mux2/3
  Mux2/1 -> Out1/1

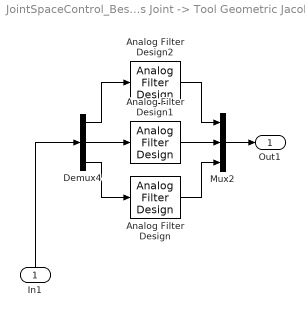
== system JointSpaceControl_BestInertia/Forward & Velocity Kinematics Joint -> Tool Geometric Jacobian/End-Effector -> Joints/Subsystem1 ==
  In1 : Inport
  Analog Filter Design : dsparch4/Analog Filter Design  method=Butterworth  filttype=Lowpass  N=8  Wlo=30  Whi=80  Rp=2  Rs=40
  Analog Filter Design1 : dsparch4/Analog Filter Design  method=Butterworth  filttype=Lowpass  N=8  Wlo=30  Whi=80  Rp=2  Rs=40
  Analog Filter Design2 : dsparch4/Analog Filter Design  method=Butterworth  filttype=Lowpass  N=8  Wlo=30  Whi=80  Rp=2  Rs=40
  Demux4 : Demux  Outputs=[1 1 1]
  Mux2 : Mux  Inputs=[1 1 1]
  Out1 : Outport
  wires:
  Mux2/1 -> Out1/1
  Analog Filter Design/1 -> Mux2/3
  Analog Filter Design1/1 -> Mux2/2
  Analog Filter Design2/1 -> Mux2/1
  Demux4/3 -> Analog Filter Design/1
  Demux4/2 -> Analog Filter Design1/1
  Demux4/1 -> Analog Filter Design2/1
  In1/1 -> Demux4/1

== system JointSpaceControl_BestInertia/Forward & Velocity Kinematics Joint -> Tool Geometric Jacobian/End-Effector -> Joints/Subsystem2 ==
  In1 : Inport
  Analog Filter Design : dsparch4/Analog Filter Design  method=Butterworth  filttype=Lowpass  N=8  Wlo=30  Whi=80  Rp=2  Rs=40
  Analog Filter Design1 : dsparch4/Analog Filter Design  method=Butterworth  filttype=Lowpass  N=8  Wlo=30  Whi=80  Rp=2  Rs=40
  Analog Filter Design2 : dsparch4/Analog Filter Design  method=Butterworth  filttype=Lowpass  N=8  Wlo=30  Whi=80  Rp=2  Rs=40
  Demux4 : Demux  Outputs=[1 1 1]
  Mux2 : Mux  Inputs=[1 1 1]
  Out1 : Outport
  wires:
  In1/1 -> Demux4/1
  Demux4/1 -> Analog Filter Design2/1
  Demux4/2 -> Analog Filter Design1/1
  Demux4/3 -> Analog Filter Design/1
  Analog Filter Design2/1 -> Mux2/1
  Analog Filter Design1/1 -> Mux2/2
  Analog Filter Design/1 -> Mux2/3
  Mux2/1 -> Out1/1

== system JointSpaceControl_BestInertia/Forward & Velocity Kinematics Joint -> Tool Geometric Jacobian/End-Effector -> Joints/Subsystem3 ==
  In1 : Inport
  Analog Filter Design3 : dsparch4/Analog Filter Design  method=Butterworth  filttype=Lowpass  N=8  Wlo=30  Whi=80  Rp=2  Rs=40
  Analog Filter Design4 : dsparch4/Analog Filter Design  method=Butterworth  filttype=Lowpass  N=8  Wlo=30  Whi=80  Rp=2  Rs=40
  Analog Filter Design5 : dsparch4/Analog Filter Design  method=Butterworth  filttype=Lowpass  N=8  Wlo=30  Whi=80  Rp=2  Rs=40
  Demux2 : Demux  Outputs=[1 1 1]
  Mux3 : Mux  Inputs=[1 1 1]
  Out1 : Outport
  wires:
  Mux3/1 -> Out1/1
  Analog Filter Design3/1 -> Mux3/3
  Demux2/3 -> Analog Filter Design3/1
  Demux2/2 -> Analog Filter Design4/1
  Analog Filter Design5/1 -> Mux3/1
  In1/1 -> Demux2/1
  Demux2/1 -> Analog Filter Design5/1
  Analog Filter Design4/1 -> Mux3/2

== matlab function JointSpaceControl_BestInertia/Inverse Dynamics M, C, g/ur5_matrices ==
  data: q input; M output; dq input; G output; CDq output
function [ M, G, CDq ] = ur5_Matrices( q, dq)
%#codegen
%Returns the acceleration of the manipulator based on its dynamics
[ M, G, CDq ] = ur5_matrices( q, dq );

== matlab function JointSpaceControl_BestInertia/Forward & Velocity Kinematics Joint -> Tool Geometric Jacobian/rank(J)1 ==
  data: J input; rank_J output
function rank_J   = rank_J(J)
%Calculate the rank of a matrix J.

rank_J = svd(J);
end

== matlab function JointSpaceControl_BestInertia/Inverse Dynamics M, C, g1/ur5_matrices ==
  data: q input; M output; dq input; G output; CDq output
function [ M, G, CDq ] = ur5_Matrices( q, dq)
%#codegen
%Returns the acceleration of the manipulator based on its dynamics
[ M, G, CDq ] = ur5_matrices( q, dq );
